simulink subsystem "Spacecraft_Dynamics"  (R2021b)
settings: Solver=VariableStepAuto  StartTime=0.0  StopTime=10.0  RelTol=1e-3
model mask{Mass=1, J=eye(3)}
  mask prompts: Mass "Mass(Kg)"; J "J(Kg*m^2)"
undefined symbols (not defined in the file): simConcifg, simConfig
settings Model: Creator=DELL  LastModifiedBy=DELL

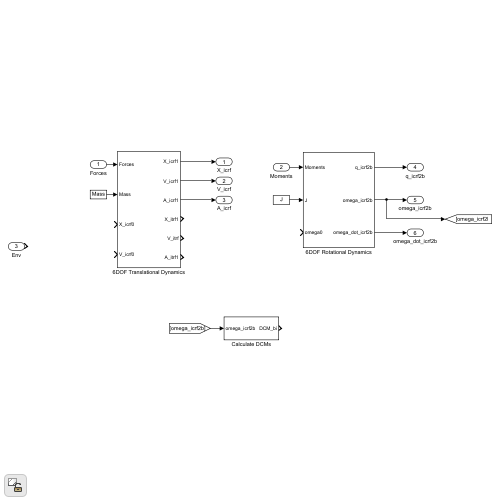
[thumbnail: Simulink's stored preview of the top-level diagram]
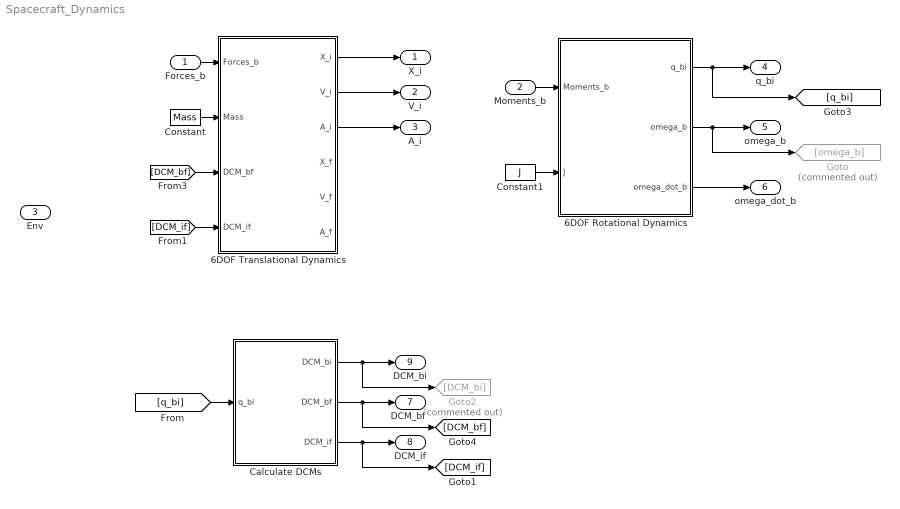
== system Spacecraft_Dynamics ==
  Forces_b : Inport
  Moments_b : Inport  Port=2
  Env : Inport  Port=3
  6DOF Rotational Dynamics : Subsystem
  6DOF Translational Dynamics : Subsystem
  Calculate DCMs : Subsystem
  Constant : Constant  Value=Mass
  Constant1 : Constant  Value=J
  Goto : Goto  Commented=on  GotoTag=omega_b
  Goto2 : Goto  Commented=on  GotoTag=DCM_bi
  X_i : Outport
  V_i : Outport  Port=2
  A_i : Outport  Port=3
  q_bi : Outport  Port=4
  omega_b : Outport  Port=5
  omega_dot_b : Outport  Port=6
  DCM_bf : Outport  Port=7
  DCM_if : Outport  Port=8
  DCM_bi : Outport  Port=9
  wires:
  6DOF Translational Dynamics/1(X_i) -> X_i/1
  6DOF Translational Dynamics/2(V_i) -> V_i/1
  6DOF Translational Dynamics/3(A_i) -> A_i/1
  Constant/1 -> 6DOF Translational Dynamics/2(Mass)
  Forces_b/1 -> 6DOF Translational Dynamics/1(Forces_b)
  Constant1/1 -> 6DOF Rotational Dynamics/2(J)
  Moments_b/1 -> 6DOF Rotational Dynamics/1(Moments_b)
  6DOF Rotational Dynamics/1(q_bi) -> q_bi/1, [q_bi]
  6DOF Rotational Dynamics/3(omega_dot_b) -> omega_dot_b/1
  6DOF Rotational Dynamics/2(omega_b) -> omega_b/1, Goto/1
  [q_bi] -> Calculate DCMs/1(q_bi)
  Calculate DCMs/3(DCM_if) -> [DCM_if], DCM_if/1
  [DCM_if] -> 6DOF Translational Dynamics/4(DCM_if)
  Calculate DCMs/1(DCM_bi) -> Goto2/1, DCM_bi/1
  Calculate DCMs/2(DCM_bf) -> [DCM_bf], DCM_bf/1
  [DCM_bf] -> 6DOF Translational Dynamics/3(DCM_bf)

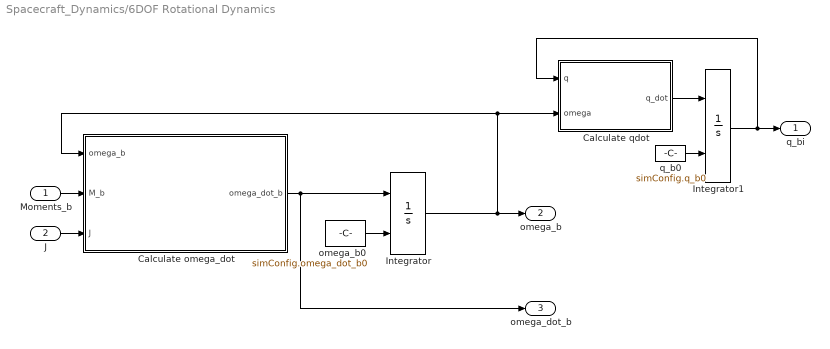
== system Spacecraft_Dynamics/6DOF Rotational Dynamics ==
  Moments_b : Inport
  J : Inport  Port=2
  Calculate omega_dot : MATLAB Function  TreatAsAtomicUnit=on
  Calculate qdot : MATLAB Function  TreatAsAtomicUnit=on
  Integrator : Integrator  InitialConditionSource=external
  Integrator1 : Integrator  InitialConditionSource=external
  omega_b0 : Constant  Value=simConfig.omega_dot_b0
  q_b0 : Constant  Value=simConfig.q_b0
  q_bi : Outport
  omega_b : Outport  Port=2
  omega_dot_b : Outport  Port=3
  wires:
  Integrator1/1 -> q_bi/1, Calculate qdot/1(q)
  q_b0/1 -> Integrator1/2
  Calculate qdot/1(q_dot) -> Integrator1/1
  omega_b0/1 -> Integrator/2
  Integrator/1 -> omega_b/1, Calculate omega_dot/1(omega_b), Calculate qdot/2(omega)
  Calculate omega_dot/1(omega_dot_b) -> omega_dot_b/1, Integrator/1
  J/1 -> Calculate omega_dot/3(J)
  Moments_b/1 -> Calculate omega_dot/2(M_b)

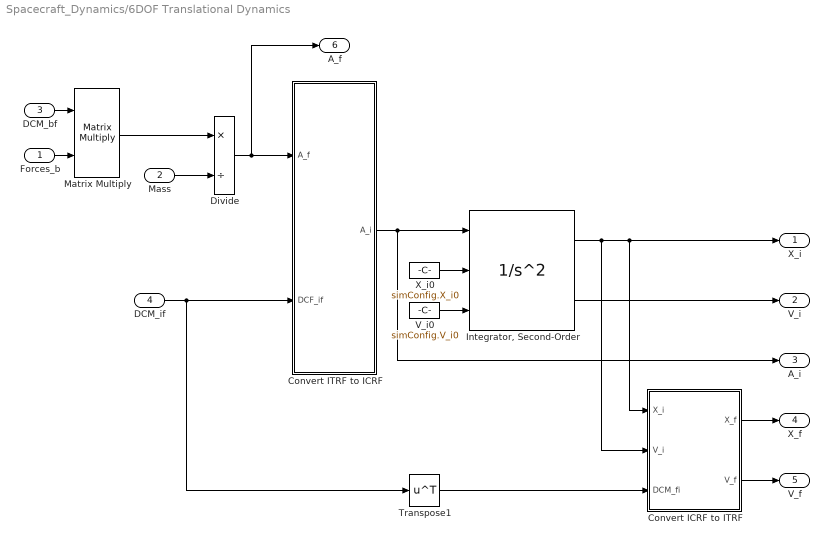
== system Spacecraft_Dynamics/6DOF Translational Dynamics ==
  Forces_b : Inport
  Mass : Inport  Port=2
  DCM_bf : Inport  Port=3
  DCM_if : Inport  Port=4
  Convert ICRF to ITRF : MATLAB Function  TreatAsAtomicUnit=on
  Convert ITRF to ICRF : MATLAB Function  TreatAsAtomicUnit=on
  Divide : Product  Inputs=*/
  "Integrator, Second-Order" : SecondOrderIntegrator  ICSourceX=external  ICSourceDXDT=external
  Matrix Multiply : Product  Multiplication=Matrix(*)
  Transpose1 : Math  Operator=transpose  SaturateOnIntegerOverflow=on
  V_i0 : Constant  Value=simConfig.V_i0
  X_i0 : Constant  Value=simConfig.X_i0
  X_i : Outport
  V_i : Outport  Port=2
  A_i : Outport  Port=3
  X_f : Outport  Port=4
  V_f : Outport  Port=5
  A_f : Outport  Port=6
  wires:
  Transpose1/1 -> Convert ICRF to ITRF/3(DCM_fi)
  Matrix Multiply/1 -> Divide/1
  Forces_b/1 -> Matrix Multiply/2
  DCM_bf/1 -> Matrix Multiply/1
  DCM_if/1 -> Transpose1/1, Convert ITRF to ICRF/2(DCF_if)
  X_i0/1 -> "Integrator, Second-Order"/2
  Divide/1 -> Convert ITRF to ICRF/1(A_f), A_f/1
  Mass/1 -> Divide/2
  V_i0/1 -> "Integrator, Second-Order"/3
  Convert ICRF to ITRF/2(V_f) -> V_f/1
  Convert ICRF to ITRF/1(X_f) -> X_f/1
  "Integrator, Second-Order"/2 -> V_i/1
  "Integrator, Second-Order"/1 -> X_i/1, Convert ICRF to ITRF/1(X_i), Convert ICRF to ITRF/2(V_i)
  Convert ITRF to ICRF/1(A_i) -> "Integrator, Second-Order"/1, A_i/1

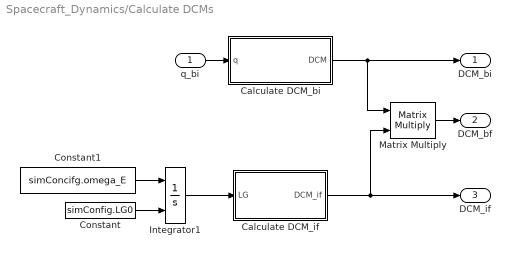
== system Spacecraft_Dynamics/Calculate DCMs ==
  q_bi : Inport
  Calculate DCM_bi : MATLAB Function  TreatAsAtomicUnit=on
  Calculate DCM_if : MATLAB Function  TreatAsAtomicUnit=on
  Constant : Constant  Value=simConfig.LG0
  Constant1 : Constant  Value=simConcifg.omega_E
  Integrator1 : Integrator  InitialConditionSource=external
  Matrix Multiply : Product  Multiplication=Matrix(*)
  DCM_bi : Outport
  DCM_bf : Outport  Port=2
  DCM_if : Outport  Port=3
  wires:
  q_bi/1 -> Calculate DCM_bi/1(q)
  Matrix Multiply/1 -> DCM_bf/1
  Calculate DCM_if/1(DCM_if) -> DCM_if/1, Matrix Multiply/2
  Integrator1/1 -> Calculate DCM_if/1(LG)
  Constant1/1 -> Integrator1/1
  Constant/1 -> Integrator1/2
  Calculate DCM_bi/1(DCM) -> DCM_bi/1, Matrix Multiply/1

== matlab function Spacecraft_Dynamics/6DOF Translational Dynamics/Convert ICRF to ITRF ==
  data: X_i input; X_f output; V_f output; V_i input; DCM_fi input
function [X_f, V_f] = fcn(X_i, V_i, DCM_fi)

X_f = DCM_fi * X_i;
V_f = DCM_fi * V_i;
end

== matlab function Spacecraft_Dynamics/6DOF Translational Dynamics/Convert ITRF to ICRF ==
  data: A_f input; A_i output; DCF_if input
function A_i  = fcn(A_f, DCF_if)

A_i = DCF_if * A_f;
end

== matlab function Spacecraft_Dynamics/6DOF Rotational Dynamics/Calculate omega_dot ==
  data: omega_b input; M_b input; omega_dot_b output; J input
function omega_dot_b = fcn(omega_b, M_b, J)

omega_dot_b = (M_b - omega_b * (J * omega_b)) / J;

== matlab function Spacecraft_Dynamics/Calculate DCMs/Calculate DCM_bi ==
  data: q input; DCM output
function DCM = fcn(q)
DCM = q2dcm(q);
end

== matlab function Spacecraft_Dynamics/Calculate DCMs/Calculate DCM_if ==
  data: LG input; DCM_if output
function DCM_if = fcn(LG)

DCM_if = lg2dcm_if(LG);
end

== matlab function Spacecraft_Dynamics/6DOF Rotational Dynamics/Calculate qdot ==
  data: q input; q_dot output; omega input
function q_dot = fcn(q, omega)
q_dot = calc_qdot(q, omega);
end
